simulink subsystem "continuous_subsys"  (R2026a)
settings: Solver=VariableStepAuto
settings Model: Creator=adam  LastModifiedBy=adam

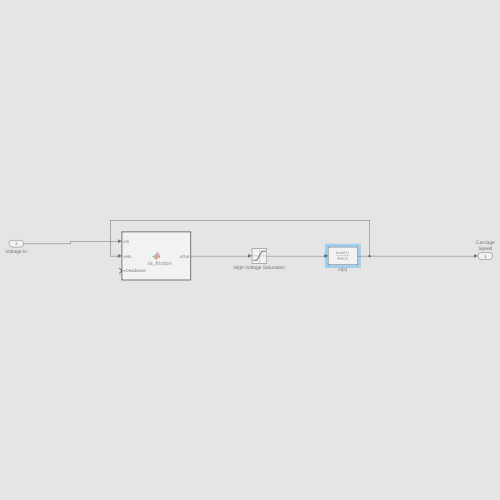
[thumbnail: Simulink's stored preview of the top-level diagram]
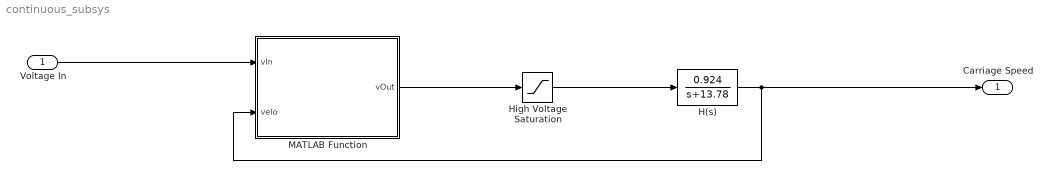
== system continuous_subsys ==
  Voltage In : Inport
  H(s) : TransferFcn  Numerator=[0.924]  Denominator=[1 13.78]
  High Voltage Saturation : Saturate  UpperLimit=35  LowerLimit=-35
  MATLAB Function : MATLAB Function  TreatAsAtomicUnit=on
  " Carriage Speed" : Outport
  wires:
  MATLAB Function/1(vOut) -> High Voltage Saturation/1
  H(s)/1 -> MATLAB Function/2(velo), " Carriage Speed"/1
  High Voltage Saturation/1 -> H(s)/1
  Voltage In/1 -> MATLAB Function/1(vIn)

== matlab function continuous_subsys/MATLAB Function ==
  data: vIn input; vOut output; velo input
function vOut = static_friction(vIn, velo)
    velo_thresh = 1e-3;

    if (abs(velo) < velo_thresh)
        voltThreshold = 1;
    else
        voltThreshold = 0.3;
    end

    if vIn > voltThreshold
        vOut = vIn - voltThreshold;
    elseif vIn < -voltThreshold
            vOut = vIn + voltThreshold;
    else
        vOut = 0;
    end
end
